simulink model "zynqRadioHWSWLTEDecimatorRFSoC2x2"  (R2022a)
settings: Solver=FixedStepDiscrete  StartTime=0.0  StopTime=2*simParams.stopTime  RelTol=1e-3
PreLoadFcn:
  | zynqRadioHWSWLTEInit;
InitFcn:
  | zynqRadioHWSWLTEInit;
values from neighbouring files (symbols this model uses):
  tb_dataIn = resample(rxWaveform,FsIn,fs)    [zynqRadioHWSWLTEInit.m]
  testWaveformData = zeros(testWaveformtableLength,1,'like',fi(0,1,16,15))    [zynqRadioHWSWLTEInit.m]
  testWaveformLength = length(testWaveform)    [zynqRadioHWSWLTEInit.m]
undefined symbols (not defined in the file or in its folder): dlDetConfig, dlDetConfig2, resample, simParams
libraries: xilinxrfsoclib x4, dspmlti4 x4, dspsrcs4 x2, simulink x2, hdlsllib x2, dspsigops x1, dsphdlfiltering2 x1
settings Model: DataTypeOverride=Off  SimulationMode=accelerator  Creator=The MathWorks, Inc.  LastModifiedBy=pshubh
settings SolverCC: AlgebraicLoopSolver=TrustRegion
settings DataIOCC: LimitDataPoints=on  SaveFormat=Array  SaveOutput=off  VisualizeSimOutput=off  SaveTime=off  ReturnWorkspaceOutputs=off
settings OptimizationCC: BlockReduction=off  BooleanDataType=off  ConditionallyExecuteInputs=off  DefaultParameterBehavior=Inlined  InheritOutputTypeSmallerThanSingle=on  EfficientMapNaN2IntZero=off  LifeSpan=inf
settings DebuggingCC: AlgebraicLoopMsg=error  SaveWithParameterizedLinksMsg=none  UnderspecifiedInitializationDetection=Classic  MergeDetectMultiDrivingBlocksExec=none  SignalResolutionControl=TryResolveAllWithWarning  InheritedTsInSrcMsg=none  SingleTaskRateTransMsg=error  ParameterPrecisionLossMsg=none  UnconnectedInputMsg=warning  UnconnectedOutputMsg=warning  UnconnectedLineMsg=warning  AllowSymbolicDim=off  StrictBusMsg=ErrorOnBusTreatedAsVector  SFUnexpectedBacktrackingDiag=warning  SFNoUnconditionalDefaultTransitionDiag=warning  SFExecutionAtInitializationDiag=none  SFMachineParentedDataDiag=warning  ArithmeticOperatorsInVariantConditions=warning
settings HardwareCC: ProdBitPerPointer=32  ProdBitPerSizeT=32  ProdBitPerPtrDiffT=32  ProdLargestAtomicFloat=None  ProdIntDivRoundTo=Undefined  ProdEndianess=Unspecified  ProdWordSize=32  ProdHWDeviceType=ASIC/FPGA->ASIC/FPGA  TargetBitPerPointer=64  TargetBitPerSizeT=64  TargetBitPerPtrDiffT=64  TargetLongLongMode=on  TargetIntDivRoundTo=Zero  TargetEndianess=LittleEndian  TargetWordSize=64  TargetHWDeviceType=MATLAB Host  ProdEqTarget=off
settings ModelReferenceCC: UpdateModelReferenceTargets=IfOutOfDate  PropagateSignalLabelsOutOfModel=off
settings SFSimCC: SimUseLocalCustomCode=off
settings RTWCC: RTWUseLocalCustomCode=off
settings CodeAppCC: MaxIdLength=128  StateflowObjectComments=on
settings GRTTargetCC: TargetLangStandard=C89/C90 (ANSI)  CombineOutputUpdateFcns=off  GRTInterface=on
settings ConfigComp: CovMetricSettings=dw  CovSaveCumulativeToWorkspaceVar=on  CovSaveSingleToWorkspaceVar=on  CovExternalEMLEnable=off  CovSFcnEnable=off

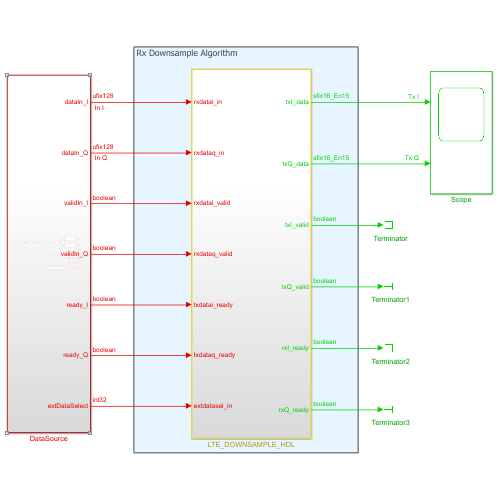
[thumbnail: Simulink's stored preview of the top-level diagram]
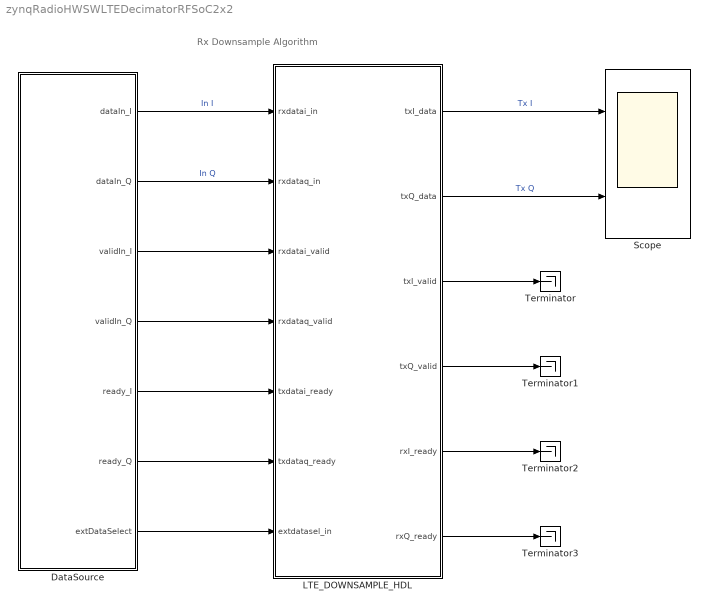
== system zynqRadioHWSWLTEDecimatorRFSoC2x2 ==
  note: Rx Downsample Algorithm
  DataSource : Subsystem
  LTE_DOWNSAMPLE_HDL : Subsystem  TreatAsAtomicUnit=on
  Scope : Scope  NumInputPorts=2
  Terminator{,1..3} (4 alike) : Terminator
  wires:
  DataSource/4(validIn_Q) -> LTE_DOWNSAMPLE_HDL/4(rxdataq_valid)
  DataSource/1(dataIn_I) -> LTE_DOWNSAMPLE_HDL/1(rxdatai_in)  "In I"
  DataSource/2(dataIn_Q) -> LTE_DOWNSAMPLE_HDL/2(rxdataq_in)  "In Q"
  DataSource/3(validIn_I) -> LTE_DOWNSAMPLE_HDL/3(rxdatai_valid)
  DataSource/7(extDataSelect) -> LTE_DOWNSAMPLE_HDL/7(extdatasel_in)
  LTE_DOWNSAMPLE_HDL/3(txI_valid) -> Terminator/1
  LTE_DOWNSAMPLE_HDL/4(txQ_valid) -> Terminator1/1
  LTE_DOWNSAMPLE_HDL/5(rxI_ready) -> Terminator2/1
  LTE_DOWNSAMPLE_HDL/6(rxQ_ready) -> Terminator3/1
  DataSource/5(ready_I) -> LTE_DOWNSAMPLE_HDL/5(txdatai_ready)
  DataSource/6(ready_Q) -> LTE_DOWNSAMPLE_HDL/6(txdataq_ready)
  LTE_DOWNSAMPLE_HDL/1(txI_data) -> Scope/1  "Tx I"
  LTE_DOWNSAMPLE_HDL/2(txQ_data) -> Scope/2  "Tx Q"

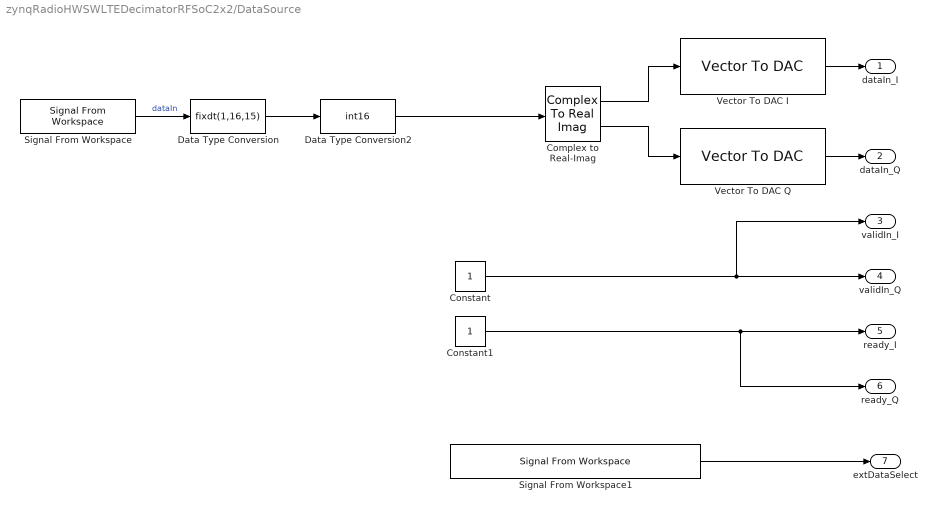
== system zynqRadioHWSWLTEDecimatorRFSoC2x2/DataSource ==
  Complex to Real-Imag : ComplexToRealImag
  Constant : Constant  VectorParams1D=off  OutDataTypeStr=boolean  SampleTime=simParams.Ts
  Constant1 : Constant  VectorParams1D=off  OutDataTypeStr=boolean  SampleTime=simParams.Ts*32
  Data Type Conversion : DataTypeConversion  OutDataTypeStr=fixdt(1,16,15)  RndMeth=Floor
  Data Type Conversion2 : DataTypeConversion  OutDataTypeStr=int16  ConvertRealWorld=Stored Integer (SI)  RndMeth=Floor
  Signal From Workspace : dspsrcs4/Signal From Workspace  X=resample(tb_dataIn,8,1)  Ts=simParams.Ts/8  nsamps=8  OutputAfterFinalValue=Cyclic repetition  ignoreOrWarnInputAndFrameLengths=on  OutputFrames=off
  Signal From Workspace1 : dspsrcs4/Signal From Workspace  X=int32([zeros(1,2457600) ones(1,3072000-2457600)])  Ts=simParams.Ts  nsamps=1  OutputAfterFinalValue=Holding final value  ignoreOrWarnInputAndFrameLengths=on  OutputFrames=off
  Vector To DAC I : xilinxrfsoclib/Vector To DAC  INPUT_WL=16  DT_INPUT=0
      settings: SourceProductBaseCode=XILINX_BLOCKSET
  Vector To DAC Q : xilinxrfsoclib/Vector To DAC  INPUT_WL=16  DT_INPUT=0
      settings: SourceProductBaseCode=XILINX_BLOCKSET
  dataIn_I : Outport
  dataIn_Q : Outport  Port=2
  validIn_I : Outport  Port=3
  validIn_Q : Outport  Port=4
  ready_I : Outport  Port=5
  ready_Q : Outport  Port=6
  extDataSelect : Outport  Port=7
  wires:
  Signal From Workspace/1 -> Data Type Conversion/1  "dataIn"
  Vector To DAC I/1 -> dataIn_I/1
  Vector To DAC Q/1 -> dataIn_Q/1
  Data Type Conversion/1 -> Data Type Conversion2/1
  Complex to Real-Imag/1 -> Vector To DAC I/1
  Complex to Real-Imag/2 -> Vector To DAC Q/1
  Signal From Workspace1/1 -> extDataSelect/1
  Constant/1 -> validIn_I/1, validIn_Q/1
  Data Type Conversion2/1 -> Complex to Real-Imag/1
  Constant1/1 -> ready_Q/1, ready_I/1

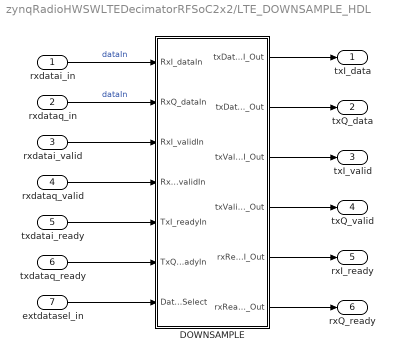
== system zynqRadioHWSWLTEDecimatorRFSoC2x2/LTE_DOWNSAMPLE_HDL ==
  rxdatai_in : Inport
  rxdataq_in : Inport  Port=2
  rxdatai_valid : Inport  Port=3
  rxdataq_valid : Inport  Port=4
  txdatai_ready : Inport  Port=5
  txdataq_ready : Inport  Port=6
  extdatasel_in : Inport  Port=7
  DOWNSAMPLE : Subsystem
  txI_data : Outport
  txQ_data : Outport  Port=2
  txI_valid : Outport  Port=3
  txQ_valid : Outport  Port=4
  rxI_ready : Outport  Port=5
  rxQ_ready : Outport  Port=6
  wires:
  DOWNSAMPLE/1(txDataI_Out) -> txI_data/1
  rxdatai_in/1 -> DOWNSAMPLE/1(RxI_dataIn)  "dataIn"
  rxdataq_in/1 -> DOWNSAMPLE/2(RxQ_dataIn)  "dataIn"
  rxdatai_valid/1 -> DOWNSAMPLE/3(RxI_validIn)
  rxdataq_valid/1 -> DOWNSAMPLE/4(RxQ_validIn)
  extdatasel_in/1 -> DOWNSAMPLE/7(Data_Select)
  DOWNSAMPLE/2(txDataQ_Out) -> txQ_data/1
  txdatai_ready/1 -> DOWNSAMPLE/5(TxI_readyIn)
  txdataq_ready/1 -> DOWNSAMPLE/6(TxQ_readyIn)
  DOWNSAMPLE/5(rxReadyI_Out) -> rxI_ready/1
  DOWNSAMPLE/6(rxReadyQ_Out) -> rxQ_ready/1
  DOWNSAMPLE/3(txValidI_Out) -> txI_valid/1
  DOWNSAMPLE/4(txValidQ_Out) -> txQ_valid/1

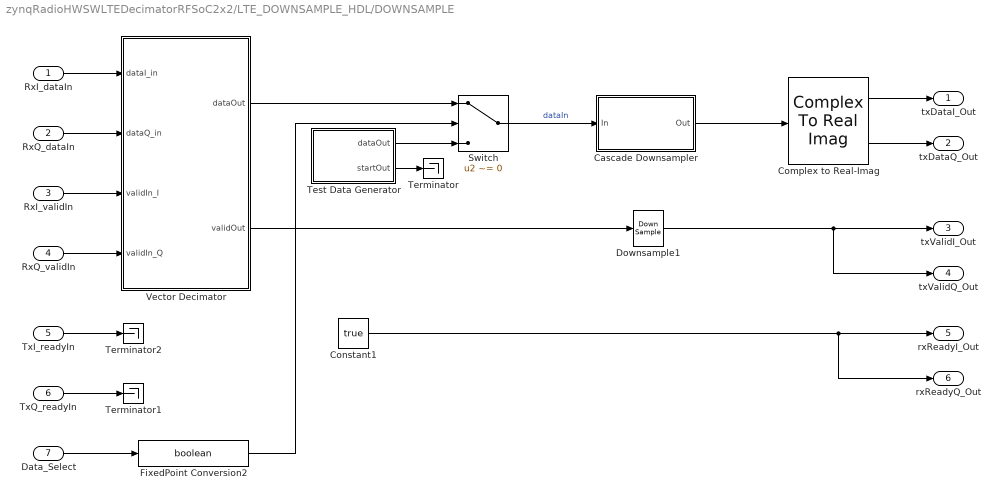
== system zynqRadioHWSWLTEDecimatorRFSoC2x2/LTE_DOWNSAMPLE_HDL/DOWNSAMPLE ==
  RxI_dataIn : Inport
  RxQ_dataIn : Inport  Port=2
  RxI_validIn : Inport  Port=3
  RxQ_validIn : Inport  Port=4
  TxI_readyIn : Inport  Port=5
  TxQ_readyIn : Inport  Port=6
  Data_Select : Inport  Port=7
  Cascade Downsampler : Subsystem
  Complex to Real-Imag : ComplexToRealImag
  Constant1 : Constant  Value=true  VectorParams1D=off  OutDataTypeStr=boolean  SampleTime=simParams.Ts
  Downsample1 : DownSample  N=32  RateOptions=Allow multirate processing
  FixedPoint Conversion2 : DataTypeConversion  OutDataTypeStr=boolean  SaturateOnIntegerOverflow=off  RndMeth=Floor
  Switch : Switch  Criteria=u2 ~= 0  SaturateOnIntegerOverflow=off  InputSameDT=off
  Terminator : Terminator
  Terminator1 : Terminator
  Terminator2 : Terminator
  Test Data Generator : Subsystem  mask{framesBetweenStarts=400}
      mask prompts: framesBetweenStarts "Number of frames between start pulses"
      mask DialogControl Control2 Prompt: (min number of frames is 2)
  Vector Decimator : Subsystem
  txDataI_Out : Outport  VectorParamsAs1DForOutWhenUnconnected=off
  txDataQ_Out : Outport  Port=2
  txValidI_Out : Outport  Port=3  VectorParamsAs1DForOutWhenUnconnected=off
  txValidQ_Out : Outport  Port=4
  rxReadyI_Out : Outport  Port=5  VectorParamsAs1DForOutWhenUnconnected=off
  rxReadyQ_Out : Outport  Port=6
  wires:
  Test Data Generator/1(dataOut) -> Switch/3
  Data_Select/1 -> FixedPoint Conversion2/1
  FixedPoint Conversion2/1 -> Switch/2
  Switch/1 -> Cascade Downsampler/1(In)  "dataIn"
  RxQ_validIn/1 -> Vector Decimator/4(validIn_Q)
  RxI_dataIn/1 -> Vector Decimator/1(dataI_in)
  RxQ_dataIn/1 -> Vector Decimator/2(dataQ_in)
  RxI_validIn/1 -> Vector Decimator/3(validIn_I)
  Vector Decimator/1(dataOut) -> Switch/1
  Cascade Downsampler/1(Out) -> Complex to Real-Imag/1
  Complex to Real-Imag/1 -> txDataI_Out/1
  Complex to Real-Imag/2 -> txDataQ_Out/1
  Test Data Generator/2(startOut) -> Terminator/1
  Vector Decimator/2(validOut) -> Downsample1/1
  TxQ_readyIn/1 -> Terminator1/1
  TxI_readyIn/1 -> Terminator2/1
  Constant1/1 -> rxReadyQ_Out/1, rxReadyI_Out/1
  Downsample1/1 -> txValidQ_Out/1, txValidI_Out/1

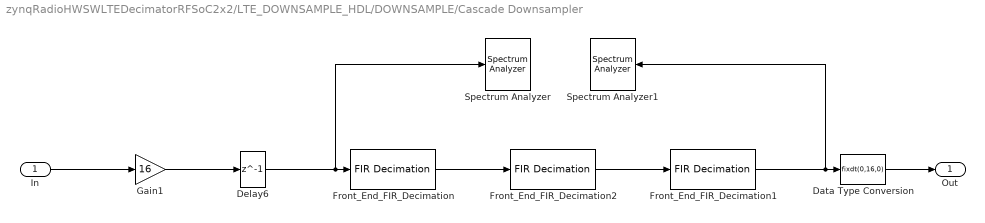
== system zynqRadioHWSWLTEDecimatorRFSoC2x2/LTE_DOWNSAMPLE_HDL/DOWNSAMPLE/Cascade Downsampler ==
  In : Inport
  Data Type Conversion : DataTypeConversion  OutDataTypeStr=fixdt(0,16,0)  ConvertRealWorld=Stored Integer (SI)  SaturateOnIntegerOverflow=off  RndMeth=Floor
  Delay6 : Delay  DelayLength=1  InitialCondition=0
  Front_End_FIR_Decimation : dspmlti4/FIR Decimation  FilterSource=Dialog parameters  h=dlDetConfig.frontEndFIRDecim.Numerator  D=dlDetConfig.frontEndFIRDecim.DecimationFactor  filtStruct=Direct form transposed  FilterObject=simParams.frontEndFIRDecim  framing=Enforce single-rate processing  inputOffset=0  outputBufInitCond=0  roundingMode=Floor  overflowMode=off  firstCoeffDataTypeStr=Inherit: Same word length as input  firstCoeffMin=[]  firstCoeffMax=[]  firstCoeffLastDataTypeStr=Inherit: Same word length as input  outputMode=Binary point scaling  outputWordLength=16  outputFracLength=15  outputDataTypeStr=fixdt(1,16,15)  outputMin=[]  outputMax=[]  outputLastDataTypeStr=fixdt(1,16,15)
      settings: LockScale=on
  Front_End_FIR_Decimation1 : dspmlti4/FIR Decimation  FilterSource=Dialog parameters  h=dlDetConfig2.frontEndFIRDecim.Numerator  D=dlDetConfig2.frontEndFIRDecim.DecimationFactor  filtStruct=Direct form transposed  FilterObject=simParams.frontEndFIRDecim  framing=Enforce single-rate processing  inputOffset=0  outputBufInitCond=0  roundingMode=Floor  overflowMode=off  firstCoeffDataTypeStr=Inherit: Same word length as input  firstCoeffMin=[]  firstCoeffMax=[]  firstCoeffLastDataTypeStr=Inherit: Same word length as input  outputMode=Binary point scaling  outputWordLength=16  outputFracLength=15  outputDataTypeStr=fixdt(1,16,15)  outputMin=[]  outputMax=[]  outputLastDataTypeStr=fixdt(1,16,15)
      settings: LockScale=on
  Front_End_FIR_Decimation2 : dspmlti4/FIR Decimation  FilterSource=Dialog parameters  h=dlDetConfig2.frontEndFIRDecim.Numerator  D=dlDetConfig2.frontEndFIRDecim.DecimationFactor  filtStruct=Direct form transposed  FilterObject=simParams.frontEndFIRDecim  framing=Enforce single-rate processing  inputOffset=0  outputBufInitCond=0  roundingMode=Floor  overflowMode=off  firstCoeffDataTypeStr=Inherit: Same word length as input  firstCoeffMin=[]  firstCoeffMax=[]  firstCoeffLastDataTypeStr=Inherit: Same word length as input  outputMode=Binary point scaling  outputWordLength=16  outputFracLength=15  outputDataTypeStr=fixdt(1,16,15)  outputMin=[]  outputMax=[]  outputLastDataTypeStr=fixdt(1,16,15)
      settings: LockScale=on
  Gain1 : Gain  Gain=16  SaturateOnIntegerOverflow=on  OutDataTypeStr=Inherit: Same as input
  Spectrum Analyzer : SpectrumAnalyzer
  Spectrum Analyzer1 : SpectrumAnalyzer
  Out : Outport
  wires:
  Gain1/1 -> Delay6/1
  In/1 -> Gain1/1
  Data Type Conversion/1 -> Out/1
  Front_End_FIR_Decimation/1 -> Front_End_FIR_Decimation2/1
  Delay6/1 -> Spectrum Analyzer/1, Front_End_FIR_Decimation/1
  Front_End_FIR_Decimation1/1 -> Spectrum Analyzer1/1, Data Type Conversion/1
  Front_End_FIR_Decimation2/1 -> Front_End_FIR_Decimation1/1

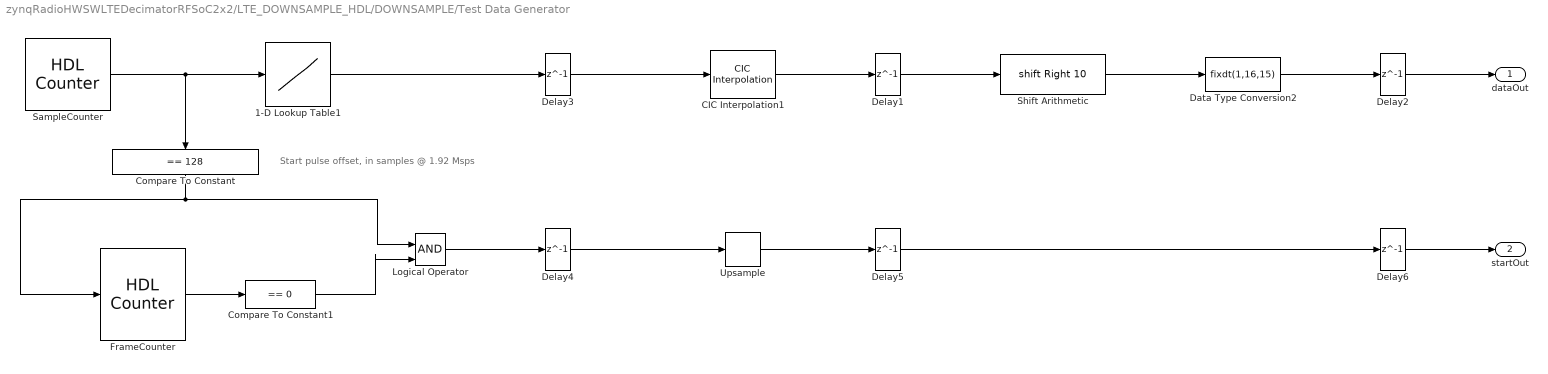
== system zynqRadioHWSWLTEDecimatorRFSoC2x2/LTE_DOWNSAMPLE_HDL/DOWNSAMPLE/Test Data Generator ==
  note: Start pulse offset, in samples @ 1.92 Msps
  1-D Lookup Table1 : Lookup_n-D  NumberOfTableDimensions=1  BreakpointsSpecification=Even spacing  BreakpointsForDimension1=[-5:5]  BreakpointsForDimension1FirstPoint=0  BreakpointsForDimension2FirstPoint=10  BreakpointsForDimension2Spacing=12  IndexSearchMethod=Evenly spaced points  Table=testWaveformData  TableDataTypeStr=testWaveformData.numerictype  InterpMethod=Flat  DiagnosticForOutOfRangeInput=Error  InternalRulePriority=Speed  OutDataTypeStr=testWaveformData.numerictype  RndMeth=Simplest
  CIC Interpolation1 : dspmlti4/CIC Interpolation  filtFrom=Dialog parameters  filtobj=Hm_interp  ftype=Interpolator  R=32  M=1  N=3  filterInternals=Full precision  BPS=[16 16 16 16]  FLPS=0  outputWordLength=32  outputFracLength=0  launchFVT=off  framing=Allow multirate processing  OutputFrames=off
      settings: SourceProductBaseCode=DS
  Compare To Constant : simulink/Logic and Bit Operations/Compare To Constant  relop===  const=128  OutDataTypeStr=boolean
  Compare To Constant1 : simulink/Logic and Bit Operations/Compare To Constant  relop===  const=0  OutDataTypeStr=boolean
  Data Type Conversion2 : DataTypeConversion  OutDataTypeStr=fixdt(1,16,15)  SaturateOnIntegerOverflow=off  RndMeth=Floor
  Delay{1..6} (6 alike) : Delay  DelayLength=1  InitialCondition=0  UseCircularBuffer=on
  FrameCounter : hdlsllib/Sources/HDL Counter  CountType=Count limited  CountInit=0  CountStep=1  CountMax=framesBetweenStarts-1  CountFromType=Initial value  CountFrom=0  CountResetPort=off  CountLoadPort=off  CountEnbPort=on  CountDirPort=off  CountHitOutputPort=off  CountDataType=Unsigned  CountWordLen=nextpow2(framesBetweenStarts)  CountFracLen=0  CountSampTime=32 * simParams.Ts
  Logical Operator : Logic  IconShape=distinctive  AllPortsSameDT=off  OutDataTypeStr=boolean
  SampleCounter : hdlsllib/Sources/HDL Counter  CountType=Count limited  CountInit=0  CountStep=1  CountMax=testWaveformLength-1  CountFromType=Initial value  CountFrom=0  CountResetPort=off  CountLoadPort=off  CountEnbPort=off  CountDirPort=off  CountHitOutputPort=off  CountDataType=Unsigned  CountWordLen=nextpow2(testWaveformLength)  CountFracLen=0  CountSampTime=32 * simParams.Ts
  Shift Arithmetic : ArithShift  BitShiftNumber=10  BitShiftDirection=Right
  Upsample : dspsigops/Upsample  N=32  phase=0  RateOptions=Allow multirate processing  ic=0  mode=Unused parameter value
  dataOut : Outport  VectorParamsAs1DForOutWhenUnconnected=off
  startOut : Outport  Port=2  VectorParamsAs1DForOutWhenUnconnected=off
  wires:
  Data Type Conversion2/1 -> Delay2/1
  CIC Interpolation1/1 -> Delay1/1
  Shift Arithmetic/1 -> Data Type Conversion2/1
  SampleCounter/1 -> 1-D Lookup Table1/1, Compare To Constant/1
  1-D Lookup Table1/1 -> Delay3/1
  Delay3/1 -> CIC Interpolation1/1
  Delay1/1 -> Shift Arithmetic/1
  Delay2/1 -> dataOut/1
  Delay4/1 -> Upsample/1
  Upsample/1 -> Delay5/1
  Delay5/1 -> Delay6/1
  Compare To Constant/1 -> Logical Operator/1, FrameCounter/1
  FrameCounter/1 -> Compare To Constant1/1
  Compare To Constant1/1 -> Logical Operator/2
  Logical Operator/1 -> Delay4/1
  Delay6/1 -> startOut/1

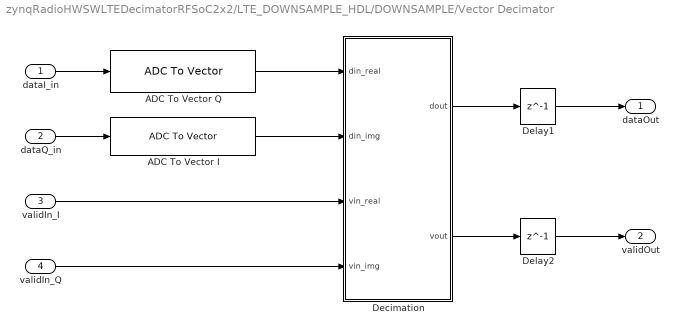
== system zynqRadioHWSWLTEDecimatorRFSoC2x2/LTE_DOWNSAMPLE_HDL/DOWNSAMPLE/Vector Decimator ==
  dataI_in : Inport
  dataQ_in : Inport  Port=2
  validIn_I : Inport  Port=3  SampleTime=1/(61.44e6)
  validIn_Q : Inport  Port=4  SampleTime=1/(61.44e6)
  ADC To Vector I : xilinxrfsoclib/ADC To Vector  samplesPerClock=8  DT=fixdt(1,16,15)  INPUT_DT=0
      settings: SourceProductBaseCode=XILINX_BLOCKSET
  ADC To Vector Q : xilinxrfsoclib/ADC To Vector  samplesPerClock=8  DT=fixdt(1,16,15)  INPUT_DT=0
      settings: SourceProductBaseCode=XILINX_BLOCKSET
  Decimation : Subsystem
  Delay1 : Delay  DelayLength=1
  Delay2 : Delay  DelayLength=1
  dataOut : Outport
  validOut : Outport  Port=2
  wires:
  validIn_Q/1 -> Decimation/4(vin_img)
  ADC To Vector Q/1 -> Decimation/1(din_real)
  ADC To Vector I/1 -> Decimation/2(din_img)
  validIn_I/1 -> Decimation/3(vin_real)
  Decimation/1(dout) -> Delay1/1
  Delay1/1 -> dataOut/1
  dataI_in/1 -> ADC To Vector Q/1
  dataQ_in/1 -> ADC To Vector I/1
  Delay2/1 -> validOut/1
  Decimation/2(vout) -> Delay2/1

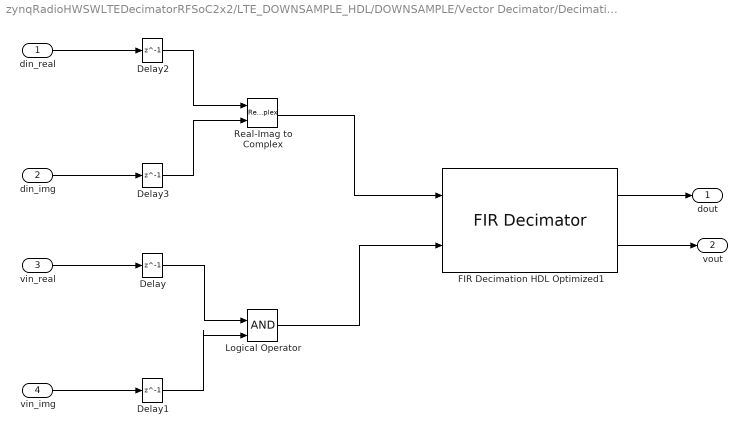
== system zynqRadioHWSWLTEDecimatorRFSoC2x2/LTE_DOWNSAMPLE_HDL/DOWNSAMPLE/Vector Decimator/Decimation ==
  din_real : Inport
  din_img : Inport  Port=2
  vin_real : Inport  Port=3
  vin_img : Inport  Port=4
  Delay{,1..3} (4 alike) : Delay  DelayLength=1  InitialCondition=0
  FIR Decimation HDL Optimized1 : dsphdlfiltering2/FIR Decimator  Numerator=fir1(35,0.4)  FilterStructure=Direct form systolic  DecimationFactor=8  NumCycles=1  SimulateUsing=Code generation  roundingMode=Floor  overflowMode=off  CoefficientsDataTypeStr=Inherit: Same word length as input  OutputDataTypeStr=fixdt(1,16,15)  ResetInputPort=off  HDLGlobalReset=off
      settings: SourceProductBaseCode=HS
  Logical Operator : Logic  IconShape=distinctive  AllPortsSameDT=off  OutDataTypeStr=boolean
  Real-Imag to Complex : RealImagToComplex
  dout : Outport  VectorParamsAs1DForOutWhenUnconnected=off
  vout : Outport  Port=2  VectorParamsAs1DForOutWhenUnconnected=off
  wires:
  FIR Decimation HDL Optimized1/1 -> dout/1
  vin_real/1 -> Delay/1
  vin_img/1 -> Delay1/1
  din_real/1 -> Delay2/1
  din_img/1 -> Delay3/1
  Real-Imag to Complex/1 -> FIR Decimation HDL Optimized1/1
  Logical Operator/1 -> FIR Decimation HDL Optimized1/2
  Delay/1 -> Logical Operator/1
  Delay1/1 -> Logical Operator/2
  Delay2/1 -> Real-Imag to Complex/1
  Delay3/1 -> Real-Imag to Complex/2
  FIR Decimation HDL Optimized1/2 -> vout/1
